simulink model "robot_controller"  (R2020b)
settings: Solver=ode45  StartTime=0.0  StopTime=10  MaxStep=0.01  RelTol=1e-3  AbsTol=1e-3  EnableMultiTasking=on
InitFcn:
  | parameters;
values from neighbouring files (symbols this model uses):
  g = 9.81    [parameters.m]
  q1_init = deg2rad(0)    [parameters.m]
  q2_init = deg2rad(0)    [parameters.m]
  q3_init = deg2rad(0)    [parameters.m]
undefined symbols (not defined in the file or in its folder): X, Y, Z
libraries: sm_lib x18, nesl_utility x13, robot_arms_library x3
settings Model: Creator=martin  LastModifiedBy=martin
settings SolverCC: AutoScaleAbsTol=off
settings DataIOCC: LimitDataPoints=on  MaxDataPoints=10000
settings OptimizationCC: LifeSpan=inf
settings DebuggingCC: AllowSymbolicDim=off  SFUnexpectedBacktrackingDiag=warning  SFNoUnconditionalDefaultTransitionDiag=warning  SFExecutionAtInitializationDiag=none  ArithmeticOperatorsInVariantConditions=warning
settings SFSimCC: SimUseLocalCustomCode=off  CustomCodeUndefinedFunction=UseInterfaceOnly
settings RTWCC: RTWUseLocalCustomCode=off
settings CodeAppCC: StateflowObjectComments=on
settings GRTTargetCC: TargetLangStandard=C89/C90 (ANSI)
settings ConfigComp: CovMetricSettings=dw  CovSaveCumulativeToWorkspaceVar=on  CovSaveSingleToWorkspaceVar=on  CovExternalEMLEnable=off  CovSFcnEnable=off
settings SimscapeCC: SimscapeLogType=all  SimscapeLogSimulationStatistics=on  SimscapeLogDataHistory=10000
settings ExplorerConfigSet: InternalSimMechanicsExplorerSettings="<ExplorerConfiguration><canonicalview>planar_xy</canonicalview><AnimationSetting><BasePlaybackSpeed>1.0</BasePlaybackSpeed><PlaybackSpeedFactor>1.0</PlaybackSpeedFactor></AnimationSetting><TilePanel><TileInfo><Tiles Columns=\"1\" Count=\"1\" Rows=\"1\"><Column Weight=\"1\"/><Row Weight=\"1\"/><Tile Height=\"1\" Width=\"1\" X=\"0\" Y=\"0\"/></Tiles></TileInfo><SceneInfo><SceneViewer><BGColor><R>0.60000002384185791</R><G>0.60000002384185791</G><B>0.60000002384185791</B></BGColor><Camera><DoPerspective>off</DoPerspective><Position><X>0.670851724377320102</X><Y>0.67664429958525496</Y><Z>0.569251006197132758</Z></Position><Center><X>0.0935014551876945238</X><Y>0.099294030395629021</Y><Z>-0.00809926299249304205</Z></Center><Up><X>-0.408248290463863073</X><Y>0.816496580927726145</Y><Z>-0.408248290463863073</Z></Up><ViewLimDist>1</ViewLimDist><YLim>0.196018997144688012</YLim><XLim>0.308076523845734696</XLim></Camera></SceneViewer></SceneInfo></TilePanel><MechEditorPanel><Cameras/><GfxPanelCameraMap/><VideoCreator><PlaybackSpeedRatio>1.0</PlaybackSpeedRatio><FrameRate>30</FrameRate><VideoFormat>Motion JPEG AVI</VideoFormat><FrameSize>[800 600]</FrameSize></VideoCreator></MechEditorPanel></ExplorerConfiguration>"

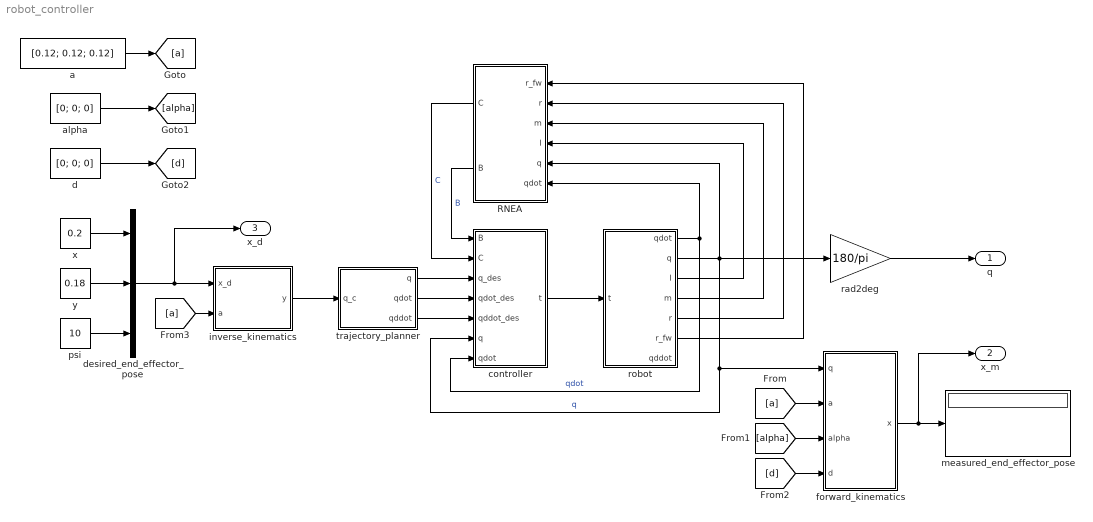
== system robot_controller ==
  RNEA : MATLAB Function  TreatAsAtomicUnit=on
  a : Constant  Value=[0.12; 0.12; 0.12]
  alpha : Constant  Value=[0; 0; 0]
  controller : Subsystem
  d : Constant  Value=[0; 0; 0]
  desired_end_effector_pose : Mux  Inputs=3
  forward_kinematics : MATLAB Function  TreatAsAtomicUnit=on
  inverse_kinematics : Subsystem
  measured_end_effector_pose : Display
  psi : Constant  Value=10
  rad2deg : Gain  Gain=180/pi
  robot : Subsystem
  trajectory_planner : Subsystem
  x : Constant  Value=0.2
  y : Constant  Value=0.18
  q : Outport
  x_m : Outport  Port=2
  x_d : Outport  Port=3
  wires:
  rad2deg/1 -> q/1
  RNEA/2(B) -> controller/1(B)  "B"
  RNEA/1(C) -> controller/2(C)  "C"
  controller/1(t) -> robot/1(t)
  trajectory_planner/1(q) -> controller/3(q_des)
  trajectory_planner/2(qdot) -> controller/4(qdot_des)
  trajectory_planner/3(qddot) -> controller/5(qddot_des)
  y/1 -> desired_end_effector_pose/2
  x/1 -> desired_end_effector_pose/1
  psi/1 -> desired_end_effector_pose/3
  desired_end_effector_pose/1 -> x_d/1, inverse_kinematics/1(x_d)
  inverse_kinematics/1(y) -> trajectory_planner/1(q_c)
  robot/2(q) -> RNEA/5(q), forward_kinematics/1(q), controller/6(q), rad2deg/1  "q"
  robot/1(qdot) -> RNEA/6(qdot), controller/7(qdot)  "qdot"
  robot/3(I) -> RNEA/4(I)
  robot/4(m) -> RNEA/3(m)
  robot/5(r) -> RNEA/2(r)
  robot/6(r_fw) -> RNEA/1(r_fw)
  a/1 -> [a]
  alpha/1 -> [alpha]
  d/1 -> [d]
  [a] -> forward_kinematics/2(a)
  [alpha] -> forward_kinematics/3(alpha)
  [d] -> forward_kinematics/4(d)
  forward_kinematics/1(x) -> x_m/1, measured_end_effector_pose/1
  [a] -> inverse_kinematics/2(a)

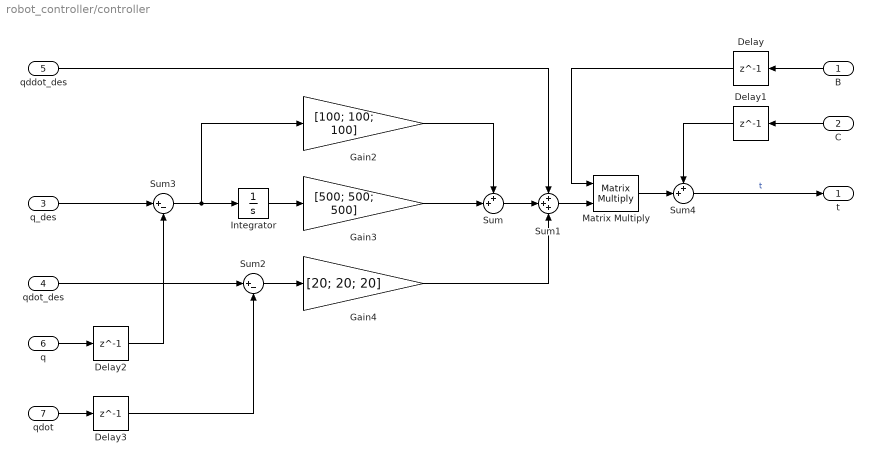
== system robot_controller/controller ==
  B : Inport
  C : Inport  Port=2
  q_des : Inport  Port=3
  qdot_des : Inport  Port=4
  qddot_des : Inport  Port=5
  q : Inport  Port=6
  qdot : Inport  Port=7
  Delay{,1..3} (4 alike) : Delay  DelayLength=1
  Gain2 : Gain  Gain=[100; 100; 100]
  Gain3 : Gain  Gain=[500; 500; 500]
  Gain4 : Gain  Gain=[20; 20; 20]
  Integrator : Integrator
  Matrix Multiply : Product  Inputs=**  Multiplication=Matrix(*)
  Sum : Sum  Inputs=++|
  Sum1 : Sum  Inputs=+++
  Sum2 : Sum  Inputs=|+-
  Sum3 : Sum  Inputs=|+-
  Sum4 : Sum  Inputs=++|
  t : Outport
  wires:
  Integrator/1 -> Gain3/1
  Sum3/1 -> Gain2/1, Integrator/1
  Sum4/1 -> t/1  "t"
  B/1 -> Delay/1
  Sum2/1 -> Gain4/1
  qdot_des/1 -> Sum2/1
  Gain2/1 -> Sum/1
  Matrix Multiply/1 -> Sum4/2
  Sum/1 -> Sum1/2
  Sum1/1 -> Matrix Multiply/2
  q_des/1 -> Sum3/1
  Gain4/1 -> Sum1/3
  qddot_des/1 -> Sum1/1
  C/1 -> Delay1/1
  Gain3/1 -> Sum/2
  q/1 -> Delay2/1
  qdot/1 -> Delay3/1
  Delay/1 -> Matrix Multiply/1
  Delay1/1 -> Sum4/1
  Delay2/1 -> Sum3/2
  Delay3/1 -> Sum2/2

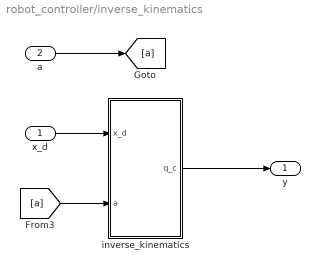
== system robot_controller/inverse_kinematics ==
  x_d : Inport
  a : Inport  Port=2
  inverse_kinematics : MATLAB Function  TreatAsAtomicUnit=on
  y : Outport
  wires:
  a/1 -> [a]
  [a] -> inverse_kinematics/2(a)
  inverse_kinematics/1(q_c) -> y/1
  x_d/1 -> inverse_kinematics/1(x_d)

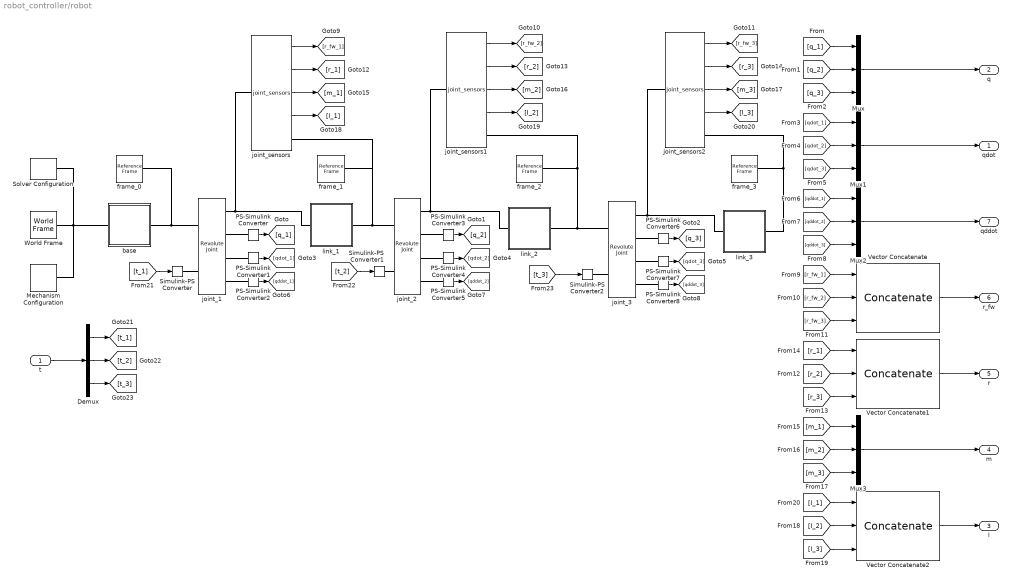
== system robot_controller/robot ==
  t : Inport
  Demux : Demux  Outputs=3
  Mechanism Configuration : sm_lib/Utilities/Mechanism Configuration  UniformGravity=Constant  GravityVector=[0 -g 0]  GravityVectorUnits=m/s^2  GravityUnits=m/s^2  LinearizationDelta=0.001  JointModeTransitionNonlinearIterations=2
      settings: SourceProductName=Multibody
  Mux{,1..3} (4 alike) : Mux  Inputs=3
  PS-Simulink Converter{,1..8} (9 alike) : nesl_utility/PS-Simulink Converter  PhysicalDomain=network_engine_domain  SubClassName=ps_output  LeftPortType=input  RightPortType=output  PseudoPeriodic=off  Frequencies=[]  Unit=inherit  AffineConversion=off
  Simulink-PS Converter : nesl_utility/Simulink-PS Converter  PhysicalDomain=network_engine_domain  SubClassName=ps_input  LeftPortType=input  RightPortType=output  PseudoPeriodic=off  Frequencies=[]  NoiseDistribution=none  NoiseParameters=[]  Unit=N*m  AffineConversion=off  FilteringAndDerivatives=provide  SimscapeFilterOrder=1  InputFilterTimeConstant=0.001  UdotUserProvided=0
  Simulink-PS Converter1 : nesl_utility/Simulink-PS Converter  PhysicalDomain=network_engine_domain  SubClassName=ps_input  LeftPortType=input  RightPortType=output  PseudoPeriodic=off  Frequencies=[]  NoiseDistribution=none  NoiseParameters=[]  Unit=N*m  AffineConversion=off  FilteringAndDerivatives=provide  SimscapeFilterOrder=1  InputFilterTimeConstant=0.001  UdotUserProvided=0
  Simulink-PS Converter2 : nesl_utility/Simulink-PS Converter  PhysicalDomain=network_engine_domain  SubClassName=ps_input  LeftPortType=input  RightPortType=output  PseudoPeriodic=off  Frequencies=[]  NoiseDistribution=none  NoiseParameters=[]  Unit=N*m  AffineConversion=off  FilteringAndDerivatives=provide  SimscapeFilterOrder=1  InputFilterTimeConstant=0.001  UdotUserProvided=0
  Solver Configuration : nesl_utility/Solver Configuration  PhysicalDomain=network_engine_domain  SubClassName=solver  LeftPortType=input  RightPortType=generic  Tones=[]  Harmonics=[]  SimulateNoise=off  Profile=off  UseLocalSampling=off  EnableSwitchedLinearOptims=on  FrequencyDomain=off  UseCCode=off  RelTol=0.001  AbsTol=1e-06  MinStep=1e-09  ToWorkspace=off  RevertToSquareIcSolve=off  NumHomotopyIterations=100  PhasorMode=off  PhasorModeNumHarmonics=1  DoDC=off  ResidualTolerance=1e-09  UseLocalSolver=off  LocalSolverChoice=NE_BACKWARD_EULER_ADVANCER  LocalSolverSampleTime=0.001  DoFixedCost=off  MaxNonlinIter=3  MaxModeIter=2  ComputeImpulses=off  ImpulseIterations=2  LinearAlgebra=Sparse  EquationFormulation=NE_TIME_EF  DelaysMemoryBudget=1024  AutomaticFiltering=on  FilteringTimeConstant=0.001  PartitionStorageMethod=AS_NEEDED  PartitionMemoryBudget=1024  PartitionMethod=FAST
      settings: SourceProductName=Utilities
  Vector Concatenate : Concatenate  NumInputs=3  Mode=Multidimensional array  ConcatenateDimension=2
  Vector Concatenate1 : Concatenate  NumInputs=3  Mode=Multidimensional array  ConcatenateDimension=2
  Vector Concatenate2 : Concatenate  NumInputs=3  Mode=Multidimensional array
  World Frame : sm_lib/Frames and Transforms/World Frame
      settings: SourceProductName=Multibody
  base : Subsystem
  frame_{0..3} (4 alike) : sm_lib/Frames and Transforms/Reference Frame
  joint_1 : sm_lib/Joints/Revolute Joint  JointMode=Normal  SenseConstraintForce=off  SenseConstraintForceX=off  SenseConstraintForceY=off  SenseConstraintForceZ=off  SenseConstraintTorque=off  SenseConstraintTorqueX=off  SenseConstraintTorqueY=off  SenseConstraintTorqueZ=off  SenseTotalForce=off  SenseTotalForceX=off  SenseTotalForceY=off  SenseTotalForceZ=off  SenseTotalTorque=off  SenseTotalTorqueX=off  SenseTotalTorqueY=off  SenseTotalTorqueZ=off  CompositeWrenchDir=FollowerOnBase  CompositeWrenchFrame=BaseFrame  EquilibriumPosition=0  EquilibriumPositionUnits=deg  SpringStiffness=0  SpringStiffnessUnits=N*m/deg  DampingCoefficient=0  DampingCoefficientUnits=N*m/(deg/s)  TorqueActuationMode=InputTorque  MotionActuationMode=ComputedMotion  SensePosition=on  SenseVelocity=on  SenseAcceleration=on  SenseTorqueForce=off  SenseLowerLimitTorqueForce=off  SenseUpperLimitTorqueForce=off  LowerLimitSpecify=off  LowerLimitBound=-90  LowerLimitBoundUnits=deg  LowerLimitStiffness=1e4  LowerLimitStiffnessUnits=N*m/deg  LowerLimitDamping=10  LowerLimitDampingUnits=N*m/(deg/s)  LowerLimitTransitionRegionWidth=0.1  LowerLimitTransitionRegionWidthUnits=deg  UpperLimitSpecify=off  UpperLimitBound=90  UpperLimitBoundUnits=deg  UpperLimitStiffness=1e4  UpperLimitStiffnessUnits=N*m/deg  UpperLimitDamping=10  UpperLimitDampingUnits=N*m/(deg/s)  UpperLimitTransitionRegionWidth=0.1  UpperLimitTransitionRegionWidthUnits=deg  PositionTargetSpecify=on  PositionTargetPriority=High  PositionTargetValue=q1_init  PositionTargetValueUnits=rad  VelocityTargetSpecify=off  VelocityTargetPriority=High  VelocityTargetValue=0  VelocityTargetValueUnits=deg/s
  joint_2 : sm_lib/Joints/Revolute Joint  JointMode=Normal  SenseConstraintForce=off  SenseConstraintForceX=off  SenseConstraintForceY=off  SenseConstraintForceZ=off  SenseConstraintTorque=off  SenseConstraintTorqueX=off  SenseConstraintTorqueY=off  SenseConstraintTorqueZ=off  SenseTotalForce=off  SenseTotalForceX=off  SenseTotalForceY=off  SenseTotalForceZ=off  SenseTotalTorque=off  SenseTotalTorqueX=off  SenseTotalTorqueY=off  SenseTotalTorqueZ=off  CompositeWrenchDir=FollowerOnBase  CompositeWrenchFrame=BaseFrame  EquilibriumPosition=0  EquilibriumPositionUnits=deg  SpringStiffness=0  SpringStiffnessUnits=N*m/deg  DampingCoefficient=0  DampingCoefficientUnits=N*m/(deg/s)  TorqueActuationMode=InputTorque  MotionActuationMode=ComputedMotion  SensePosition=on  SenseVelocity=on  SenseAcceleration=on  SenseTorqueForce=off  SenseLowerLimitTorqueForce=off  SenseUpperLimitTorqueForce=off  LowerLimitSpecify=off  LowerLimitBound=-90  LowerLimitBoundUnits=deg  LowerLimitStiffness=1e4  LowerLimitStiffnessUnits=N*m/deg  LowerLimitDamping=10  LowerLimitDampingUnits=N*m/(deg/s)  LowerLimitTransitionRegionWidth=0.1  LowerLimitTransitionRegionWidthUnits=deg  UpperLimitSpecify=off  UpperLimitBound=90  UpperLimitBoundUnits=deg  UpperLimitStiffness=1e4  UpperLimitStiffnessUnits=N*m/deg  UpperLimitDamping=10  UpperLimitDampingUnits=N*m/(deg/s)  UpperLimitTransitionRegionWidth=0.1  UpperLimitTransitionRegionWidthUnits=deg  PositionTargetSpecify=on  PositionTargetPriority=High  PositionTargetValue=q2_init  PositionTargetValueUnits=rad  VelocityTargetSpecify=off  VelocityTargetPriority=High  VelocityTargetValue=0  VelocityTargetValueUnits=deg/s
  joint_3 : sm_lib/Joints/Revolute Joint  JointMode=Normal  SenseConstraintForce=off  SenseConstraintForceX=off  SenseConstraintForceY=off  SenseConstraintForceZ=off  SenseConstraintTorque=off  SenseConstraintTorqueX=off  SenseConstraintTorqueY=off  SenseConstraintTorqueZ=off  SenseTotalForce=off  SenseTotalForceX=off  SenseTotalForceY=off  SenseTotalForceZ=off  SenseTotalTorque=off  SenseTotalTorqueX=off  SenseTotalTorqueY=off  SenseTotalTorqueZ=off  CompositeWrenchDir=FollowerOnBase  CompositeWrenchFrame=BaseFrame  EquilibriumPosition=0  EquilibriumPositionUnits=deg  SpringStiffness=0  SpringStiffnessUnits=N*m/deg  DampingCoefficient=0  DampingCoefficientUnits=N*m/(deg/s)  TorqueActuationMode=InputTorque  MotionActuationMode=ComputedMotion  SensePosition=on  SenseVelocity=on  SenseAcceleration=on  SenseTorqueForce=off  SenseLowerLimitTorqueForce=off  SenseUpperLimitTorqueForce=off  LowerLimitSpecify=off  LowerLimitBound=-90  LowerLimitBoundUnits=deg  LowerLimitStiffness=1e4  LowerLimitStiffnessUnits=N*m/deg  LowerLimitDamping=10  LowerLimitDampingUnits=N*m/(deg/s)  LowerLimitTransitionRegionWidth=0.1  LowerLimitTransitionRegionWidthUnits=deg  UpperLimitSpecify=off  UpperLimitBound=90  UpperLimitBoundUnits=deg  UpperLimitStiffness=1e4  UpperLimitStiffnessUnits=N*m/deg  UpperLimitDamping=10  UpperLimitDampingUnits=N*m/(deg/s)  UpperLimitTransitionRegionWidth=0.1  UpperLimitTransitionRegionWidthUnits=deg  PositionTargetSpecify=on  PositionTargetPriority=High  PositionTargetValue=q3_init  PositionTargetValueUnits=rad  VelocityTargetSpecify=off  VelocityTargetPriority=High  VelocityTargetValue=0  VelocityTargetValueUnits=deg/s
  joint_sensors : robot_arms_library/joint_sensors  SystemSampleTime=-1  VariantActivationTime=update diagram  Latency=0  AutoFrameSizeCalculation=off
  joint_sensors1 : robot_arms_library/joint_sensors  SystemSampleTime=-1  VariantActivationTime=update diagram  Latency=0  AutoFrameSizeCalculation=off
  joint_sensors2 : robot_arms_library/joint_sensors  SystemSampleTime=-1  VariantActivationTime=update diagram  Latency=0  AutoFrameSizeCalculation=off
  link_1 : Subsystem
  link_2 : Subsystem
  link_3 : Subsystem
  qdot : Outport  PortDimensions=[3,1]
  q : Outport  Port=2  PortDimensions=[3,1]
  I : Outport  Port=3
  m : Outport  Port=4
  r : Outport  Port=5
  r_fw : Outport  Port=6
  qddot : Outport  Port=7  PortDimensions=[3,1]
  wires:
  [qddot_2] -> Mux2/2
  joint_sensors1/3 -> [m_2]
  [r_2] -> Vector Concatenate1/2
  PS-Simulink Converter6/1 -> [q_3]
  [qddot_3] -> Mux2/3
  [I_2] -> Vector Concatenate2/2
  t/1 -> Demux/1
  [qdot_3] -> Mux1/3
  [t_3] -> Simulink-PS Converter2/1
  PS-Simulink Converter1/1 -> [qdot_1]
  Vector Concatenate/1 -> r_fw/1
  Mux/1 -> q/1
  [r_fw_1] -> Vector Concatenate/1
  Demux/2 -> [t_2]
  joint_sensors2/4 -> [I_3]
  Vector Concatenate2/1 -> I/1
  joint_sensors/4 -> [I_1]
  Mux2/1 -> qddot/1
  [m_1] -> Mux3/1
  joint_sensors/2 -> [r_1]
  [t_2] -> Simulink-PS Converter1/1
  Mux1/1 -> qdot/1
  PS-Simulink Converter/1 -> [q_1]
  Demux/3 -> [t_3]
  joint_sensors/3 -> [m_1]
  Demux/1 -> [t_1]
  [r_fw_2] -> Vector Concatenate/2
  joint_sensors/1 -> [r_fw_1]
  [q_1] -> Mux/1
  [t_1] -> Simulink-PS Converter/1
  PS-Simulink Converter4/1 -> [qdot_2]
  PS-Simulink Converter2/1 -> [qddot_1]
  joint_sensors1/1 -> [r_fw_2]
  joint_sensors2/1 -> [r_fw_3]
  PS-Simulink Converter7/1 -> [qdot_3]
  [m_3] -> Mux3/3
  [r_1] -> Vector Concatenate1/1
  joint_sensors1/4 -> [I_2]
  [r_fw_3] -> Vector Concatenate/3
  joint_sensors1/2 -> [r_2]
  PS-Simulink Converter8/1 -> [qddot_3]
  [r_3] -> Vector Concatenate1/3
  [q_2] -> Mux/2
  [q_3] -> Mux/3
  PS-Simulink Converter3/1 -> [q_2]
  [I_1] -> Vector Concatenate2/1
  Vector Concatenate1/1 -> r/1
  [m_2] -> Mux3/2
  joint_sensors2/2 -> [r_3]
  [qddot_1] -> Mux2/1
  Mux3/1 -> m/1
  [qdot_1] -> Mux1/1
  joint_sensors2/3 -> [m_3]
  [I_3] -> Vector Concatenate2/3
  [qdot_2] -> Mux1/2
  PS-Simulink Converter5/1 -> [qddot_2]
  connections:
  joint_3/RConn4 -- PS-Simulink Converter8/LConn1
  Simulink-PS Converter/RConn1 -- joint_1/LConn2
  joint_1/RConn3 -- PS-Simulink Converter1/LConn1
  joint_1/RConn4 -- PS-Simulink Converter2/LConn1
  Simulink-PS Converter2/RConn1 -- joint_3/LConn2
  link_1/LConn1 -- joint_sensors/LConn1 -- joint_1/RConn1
  link_2/LConn1 -- joint_sensors1/LConn1 -- joint_2/RConn1
  PS-Simulink Converter6/LConn1 -- joint_3/RConn2
  joint_sensors1/RConn1 -- frame_2/RConn1 -- link_2/RConn1 -- joint_3/LConn1
  Mechanism Configuration/RConn1 -- World Frame/RConn1 -- base/LConn1 -- Solver Configuration/RConn1
  frame_3/RConn1 -- joint_sensors2/RConn1 -- link_3/RConn1
  frame_0/RConn1 -- base/RConn1 -- joint_1/LConn1
  joint_3/RConn3 -- PS-Simulink Converter7/LConn1
  joint_2/RConn4 -- PS-Simulink Converter5/LConn1
  PS-Simulink Converter/LConn1 -- joint_1/RConn2
  Simulink-PS Converter1/RConn1 -- joint_2/LConn2
  joint_2/RConn3 -- PS-Simulink Converter4/LConn1
  joint_2/LConn1 -- joint_sensors/RConn1 -- frame_1/RConn1 -- link_1/RConn1
  link_3/LConn1 -- joint_sensors2/LConn1 -- joint_3/RConn1
  PS-Simulink Converter3/LConn1 -- joint_2/RConn2

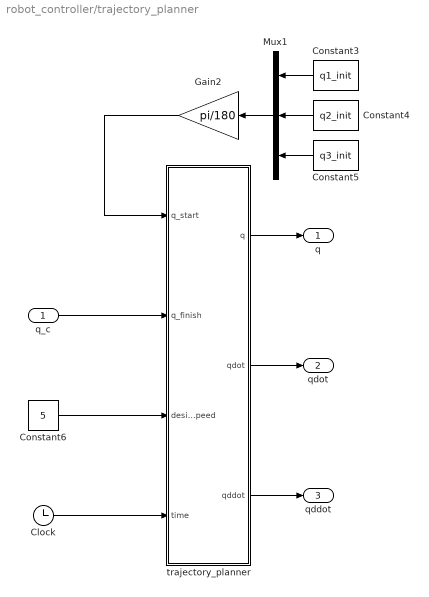
== system robot_controller/trajectory_planner ==
  q_c : Inport
  Clock : Clock
  Constant3 : Constant  Value=q1_init
  Constant4 : Constant  Value=q2_init
  Constant5 : Constant  Value=q3_init
  Constant6 : Constant  Value=5
  Gain2 : Gain  Gain=pi/180
  Mux1 : Mux  Inputs=3
  trajectory_planner : MATLAB Function  TreatAsAtomicUnit=on
  q : Outport
  qdot : Outport  Port=2
  qddot : Outport  Port=3
  wires:
  Constant6/1 -> trajectory_planner/3(desired_speed)
  Clock/1 -> trajectory_planner/4(time)
  Mux1/1 -> Gain2/1
  trajectory_planner/3(qddot) -> qddot/1
  Constant3/1 -> Mux1/1
  Constant5/1 -> Mux1/3
  trajectory_planner/2(qdot) -> qdot/1
  trajectory_planner/1(q) -> q/1
  q_c/1 -> trajectory_planner/2(q_finish)
  Gain2/1 -> trajectory_planner/1(q_start)
  Constant4/1 -> Mux1/2

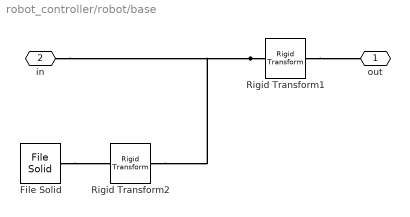
== system robot_controller/robot/base ==
  File Solid : sm_lib/Body Elements/File Solid  ExtGeomFileName=/home/martin/robot_arms/three_link_planar_arm/STEP/base.step  UnitType=FromFile  ExtGeomFileUnits=m  StepReaderType=HEX  ExportConvexHullGeometry=off  InertiaType=CalculateFromGeometry  Mass=1  MassUnits=kg  CenterOfMass=[0 0 0]  CenterOfMassUnits=m  MomentsOfInertia=[1 1 1]  MomentsOfInertiaUnits=kg*m^2  ProductsOfInertia=[0 0 0]  ProductsOfInertiaUnits=kg*m^2  BasedOnType=Density  Density=steel_density  DensityUnits=kg/m^3  DoExposeReferenceFrame=on  SerializedFrames=<Frames/>  GraphicType=FromGeometry  MarkerShape=Sphere  MarkerSize=10  GraphicVisPropType=SimpleVisualProperties  GraphicDiffuseColor=[0.5 0.5 0.5]  GraphicSpecularColor=[0.5 0.5 0.5 1.0]  GraphicAmbientColor=[0.15 0.15 0.15 1.0]  GraphicEmissiveColor=[0.0 0.0 0.0 1.0]  GraphicShininess=75  GraphicOpacity=1.0
  Rigid Transform1 : sm_lib/Frames and Transforms/Rigid Transform  TranslationMethod=StandardAxis  TranslationStandardOffset=35  TranslationLengthUnit=mm  TranslationStandardAxis=+Y  TranslationCartesianOffset=[0 0 0]  TranslationROffset=0  TranslationROffsetUnits=m  TranslationZOffset=0  TranslationZOffsetUnits=m  TranslationThetaOffset=0  TranslationThetaOffsetUnits=deg  RotationMethod=None  RotationAngleUnits=deg  RotationStandardAxis=+Z  RotationAngle=0.0  RotationArbitraryAxis=[0 0 1]  FollAlignAxisA=+X  BaseAlignAxisA=+Y  FollAlignAxisB=+Y  BaseAlignAxisB=+Z  RotationSequenceAxes=FollowerAxes  RotationSequence=XYX  RotationSequenceAngles=[0 0 0]  RotationSequenceAnglesUnits=deg  RotationMatrix=[1 0 0; 0 1 0; 0 0 1]
  Rigid Transform2 : sm_lib/Frames and Transforms/Rigid Transform  TranslationMethod=None  TranslationStandardOffset=0  TranslationLengthUnit=m  TranslationStandardAxis=+Z  TranslationCartesianOffset=[0 0 0]  TranslationROffset=0  TranslationROffsetUnits=m  TranslationZOffset=0  TranslationZOffsetUnits=m  TranslationThetaOffset=0  TranslationThetaOffsetUnits=deg  RotationMethod=StandardAxis  RotationAngleUnits=deg  RotationStandardAxis=+X  RotationAngle=90  RotationArbitraryAxis=[0 0 1]  FollAlignAxisA=+X  BaseAlignAxisA=+Y  FollAlignAxisB=+Y  BaseAlignAxisB=+Z  RotationSequenceAxes=FollowerAxes  RotationSequence=XYX  RotationSequenceAngles=[0 0 0]  RotationSequenceAnglesUnits=deg  RotationMatrix=[1 0 0; 0 1 0; 0 0 1]
  out : PMIOPort  Side=Right
  in : PMIOPort  Port=2  Side=Left
  connections:
  Rigid Transform1/LConn1 -- in/RConn1 -- Rigid Transform2/RConn1
  Rigid Transform1/RConn1 -- out/RConn1
  File Solid/RConn1 -- Rigid Transform2/LConn1

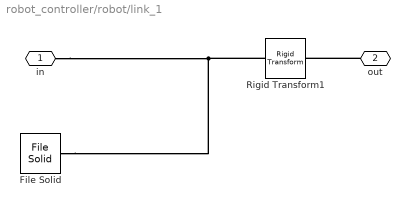
== system robot_controller/robot/link_1 ==
  File Solid : sm_lib/Body Elements/File Solid  ExtGeomFileName=/home/martin/robot_arms/three_link_planar_arm/STEP/link_1.step  UnitType=FromFile  ExtGeomFileUnits=m  StepReaderType=HEX  ExportConvexHullGeometry=off  InertiaType=CalculateFromGeometry  Mass=1  MassUnits=kg  CenterOfMass=[0 0 0]  CenterOfMassUnits=m  MomentsOfInertia=[1 1 1]  MomentsOfInertiaUnits=kg*m^2  ProductsOfInertia=[0 0 0]  ProductsOfInertiaUnits=kg*m^2  BasedOnType=Density  Density=aluminium_density  DensityUnits=kg/m^3  DoExposeReferenceFrame=on  SerializedFrames=<Frames/>  GraphicType=FromGeometry  MarkerShape=Sphere  MarkerSize=10  GraphicVisPropType=SimpleVisualProperties  GraphicDiffuseColor=[0.0 0.4 1.0]  GraphicSpecularColor=[0.5 0.5 0.5 1.0]  GraphicAmbientColor=[0.15 0.15 0.15 1.0]  GraphicEmissiveColor=[0.0 0.0 0.0 1.0]  GraphicShininess=75  GraphicOpacity=1.0
  Rigid Transform1 : sm_lib/Frames and Transforms/Rigid Transform  TranslationMethod=StandardAxis  TranslationStandardOffset=120  TranslationLengthUnit=mm  TranslationStandardAxis=+X  TranslationCartesianOffset=[0 0 0]  TranslationROffset=0  TranslationROffsetUnits=m  TranslationZOffset=0  TranslationZOffsetUnits=m  TranslationThetaOffset=0  TranslationThetaOffsetUnits=deg  RotationMethod=None  RotationAngleUnits=deg  RotationStandardAxis=+Z  RotationAngle=0.0  RotationArbitraryAxis=[0 0 1]  FollAlignAxisA=+X  BaseAlignAxisA=+Y  FollAlignAxisB=+Y  BaseAlignAxisB=+Z  RotationSequenceAxes=FollowerAxes  RotationSequence=XYX  RotationSequenceAngles=[0 0 0]  RotationSequenceAnglesUnits=deg  RotationMatrix=[1 0 0; 0 1 0; 0 0 1]
  in : PMIOPort  Side=Left
  out : PMIOPort  Port=2  Side=Right
  connections:
  out/RConn1 -- Rigid Transform1/RConn1
  Rigid Transform1/LConn1 -- in/RConn1 -- File Solid/RConn1

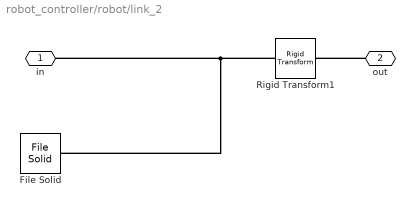
== system robot_controller/robot/link_2 ==
  File Solid : sm_lib/Body Elements/File Solid  ExtGeomFileName=/home/martin/robot_arms/three_link_planar_arm/STEP/link_2.step  UnitType=FromFile  ExtGeomFileUnits=m  StepReaderType=HEX  ExportConvexHullGeometry=off  InertiaType=CalculateFromGeometry  Mass=1  MassUnits=kg  CenterOfMass=[0 0 0]  CenterOfMassUnits=m  MomentsOfInertia=[1 1 1]  MomentsOfInertiaUnits=kg*m^2  ProductsOfInertia=[0 0 0]  ProductsOfInertiaUnits=kg*m^2  BasedOnType=Density  Density=aluminium_density  DensityUnits=kg/m^3  DoExposeReferenceFrame=on  SerializedFrames=<Frames/>  GraphicType=FromGeometry  MarkerShape=Sphere  MarkerSize=10  GraphicVisPropType=SimpleVisualProperties  GraphicDiffuseColor=[1.0 0.8 0.0]  GraphicSpecularColor=[0.5 0.5 0.5 1.0]  GraphicAmbientColor=[0.15 0.15 0.15 1.0]  GraphicEmissiveColor=[0.0 0.0 0.0 1.0]  GraphicShininess=75  GraphicOpacity=1.0
  Rigid Transform1 : sm_lib/Frames and Transforms/Rigid Transform  TranslationMethod=StandardAxis  TranslationStandardOffset=120  TranslationLengthUnit=mm  TranslationStandardAxis=+X  TranslationCartesianOffset=[0 0 0]  TranslationROffset=0  TranslationROffsetUnits=m  TranslationZOffset=0  TranslationZOffsetUnits=m  TranslationThetaOffset=0  TranslationThetaOffsetUnits=deg  RotationMethod=None  RotationAngleUnits=deg  RotationStandardAxis=+Z  RotationAngle=0.0  RotationArbitraryAxis=[0 0 1]  FollAlignAxisA=+X  BaseAlignAxisA=+Y  FollAlignAxisB=+Y  BaseAlignAxisB=+Z  RotationSequenceAxes=FollowerAxes  RotationSequence=XYX  RotationSequenceAngles=[0 0 0]  RotationSequenceAnglesUnits=deg  RotationMatrix=[1 0 0; 0 1 0; 0 0 1]
  in : PMIOPort  Side=Left
  out : PMIOPort  Port=2  Side=Right
  connections:
  out/RConn1 -- Rigid Transform1/RConn1
  Rigid Transform1/LConn1 -- in/RConn1 -- File Solid/RConn1

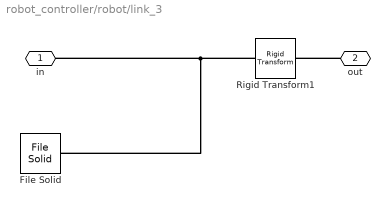
== system robot_controller/robot/link_3 ==
  File Solid : sm_lib/Body Elements/File Solid  ExtGeomFileName=/home/martin/robot_arms/three_link_planar_arm/STEP/link_3.step  UnitType=FromFile  ExtGeomFileUnits=m  StepReaderType=HEX  ExportConvexHullGeometry=off  InertiaType=CalculateFromGeometry  Mass=1  MassUnits=kg  CenterOfMass=[0 0 0]  CenterOfMassUnits=m  MomentsOfInertia=[1 1 1]  MomentsOfInertiaUnits=kg*m^2  ProductsOfInertia=[0 0 0]  ProductsOfInertiaUnits=kg*m^2  BasedOnType=Density  Density=aluminium_density  DensityUnits=kg/m^3  DoExposeReferenceFrame=on  SerializedFrames=<Frames/>  GraphicType=FromGeometry  MarkerShape=Sphere  MarkerSize=10  GraphicVisPropType=SimpleVisualProperties  GraphicDiffuseColor=[1.0 0.0 0.2]  GraphicSpecularColor=[0.5 0.5 0.5 1.0]  GraphicAmbientColor=[0.15 0.15 0.15 1.0]  GraphicEmissiveColor=[0.0 0.0 0.0 1.0]  GraphicShininess=75  GraphicOpacity=1.0
  Rigid Transform1 : sm_lib/Frames and Transforms/Rigid Transform  TranslationMethod=StandardAxis  TranslationStandardOffset=120  TranslationLengthUnit=mm  TranslationStandardAxis=+X  TranslationCartesianOffset=[0 0 0]  TranslationROffset=0  TranslationROffsetUnits=m  TranslationZOffset=0  TranslationZOffsetUnits=m  TranslationThetaOffset=0  TranslationThetaOffsetUnits=deg  RotationMethod=None  RotationAngleUnits=deg  RotationStandardAxis=+Z  RotationAngle=0.0  RotationArbitraryAxis=[0 0 1]  FollAlignAxisA=+X  BaseAlignAxisA=+Y  FollAlignAxisB=+Y  BaseAlignAxisB=+Z  RotationSequenceAxes=FollowerAxes  RotationSequence=XYX  RotationSequenceAngles=[0 0 0]  RotationSequenceAnglesUnits=deg  RotationMatrix=[1 0 0; 0 1 0; 0 0 1]
  in : PMIOPort  Side=Left
  out : PMIOPort  Port=2  Side=Right
  connections:
  Rigid Transform1/LConn1 -- in/RConn1 -- File Solid/RConn1
  out/RConn1 -- Rigid Transform1/RConn1

== matlab function robot_controller/inverse_kinematics/inverse_kinematics ==
  data: x_d input; a input; q_c output
function q_c = fcn(x_d, a)
q_c = three_link_planar_arm_IK(x_d, a);

== matlab function robot_controller/trajectory_planner/trajectory_planner ==
  data: q_start input; q output; qdot output; qddot output; q_finish input; desired_speed input; time input
function [q, qdot, qddot] = fcn(q_start, q_finish, desired_speed, time)
n = length(q_start);

q_diff = abs(q_start - q_finish);
q_max = max(q_diff);
time_taken = q_max/((pi/30)*desired_speed);
speeds = zeros(n,1);
    
    for i = 1:1:n
        if q_diff(i,1) == q_max
            speeds(i,1) = desired_speed;
        else
            speeds(i,1) = (30/pi)*q_diff(i,1)/time_taken;
        end
    end

q = zeros(n,1);
qdot = zeros(n,1);
qddot = zeros(n,1);

    for i = 1:1:n
        s = motion_planner(q_start(i,1), q_finish(i,1), speeds(i,1), 1e-02);
        if time > s.time_final
            q(i,1) = q_finish(i,1);
            qdot(i,1) = 0;
            qddot(i,1) = 0;
        else
            [q(i,1), qdot(i,1), qddot(i,1)] = s.generate_trajectory(time);
        end
    end
end

== matlab function robot_controller/RNEA ==
  data: r_fw input; r input; m input; I input; q input; qdot input; C output size=[3,1]; B output size=[3,3]; g parameter
function [C, B] = fcn(r_fw, r, m, I, q, qdot, g)
r_bw = r_fw;
pddot_init = [0; g; 0];
alpha = zeros(3,1);
kr = ones(3,1);
zm = [zeros(2,3); ones(1,3)];
Im = zeros(3,1);
joint_type = ['r'; 'r'; 'r'];
s = RNEA(joint_type, q, alpha, r, r_bw, kr, zm, m, I, Im);
[B, C] = s.dynamic_matrices(qdot, pddot_init);
end

== matlab function robot_controller/forward_kinematics ==
  data: q input; x output; a input; alpha input; d input
function x = fcn(q, a, alpha, d)
joint_type = ['r'; 'r'; 'r'];
s = forward_kinematics(joint_type, q, a, alpha, d);
x_m = s.end_effector_pose();
x = [x_m(1:2,:); (180/pi)*x_m(6,:)];
